simulink model "HouseExampleGood"  (R2023b)
settings: Solver=VariableStepAuto  StartTime=0.0  StopTime=3600*50  FixedStep=1  RelTol=1e-3  AbsTol=1e-3  EnableMultiTasking=on
PreLoadFcn:
  | % Walls
  | lenHouse   = 30;          % House length [m]
  | widHouse   = 10;          % House width [m]
  | htHouse     = 4;            % House height [m]
  | LWall           = 0.2;         % Wall thickness [m]
  | wallDensity = 1920;      % Density [kg/m^3]
  | c_wall          = 835;        % Specific heat [J/kg/K]
  | kWall            = 0.038;    % Thermal conductivity [W/m/K]
  | 
  | % Windows
  | n1_window       = 3;          % Number or windows in room 1
  | n2_window       = 2;          % Number or windows in room 2
  | n3_window       = 2;          % Number or windows in room 3
  | n4_window       = 2;          % Number or windows in room 4
  | htWindows       = 1;          % Height of windows [m]
  | widWindows      = 1;          % Width of windows  [m]
  | LWindow           = 0.01;     % Thickenss of windows [m]
  | windowDensity = 2700;    % Density [kg/m^3]
  | c_window          = 840;      % Specific heat [J/kg/K]
  | kWindow           = 0.78;     % Thermal conductivity [W/m/K]
  | 
  | 
  | % Roof
  | pitRoof         = 40/180/pi;   % Roof pitch (40 deg)
  | LRoof           = 0.2;             % Roof thickness [m]
  | roofDensity = 32;              % Roof density (Glass fiber) [kg/m^3]
  | c_roof          = 835;            % Specific heat [J/kg/K]
  | kRoof           = 0.038;         % Thermal conductivity [W/m/K]
  | 
  | % Radiators
  | %% Exchange area with air
  | S_radiator1 = 5;     % [m^2]
  | S_radiator2 = 5;     % [m^2]
  | S_radiator3 = 5;     % [m^2]
  | S_radiator4 = 5;     % [m^2]
  | %% Convective heat transfer coefficient radiator -> room
  | h_radiator1 = 100;  %  [W/(m^2 * K)]
  | h_radiator2 = 100;  %  [W/(m^2 * K)]
  | h_radiator3 = 100;  %  [W/(m^2 * K)]
  | h_radiator4 = 100;  %  [W/(m^2 * K)]
  | 
  | % Convective heat transfer coefficients [W/M^2/K]
  | h_air_wall         = 24;    % Indoor air->walls
  | h_wall_atm       = 34;   % Walls -> atmosphere
  | h_air_window    = 25;   % Indoor air -> windows
  | h_window_atm = 32;    % Windows -> atmosphere
  | h_air_roof         = 12;   % Indoor air -> roof
  | h_roof_atm      = 38;    % Roof -> atmosphere
  | 
  | %Air
  | c_air = 1005.4;         % cp of air at 273 K [J/(kg*K]
  | 
  | % Leakage fraction
  | leak_roof_percent = 0.1;     % Leakage through roof
  | leak_wall_percent  = 0.15;  % Leakage through walls
  | leak_win_percent  = 0.2;     % Leakage through windows
InitFcn:
  | % Roof
  | roofArea =  2* (widHouse/(2*cos(pitRoof))*lenHouse);
  | 
  | %Rooms
  | %% Room 1
  | area_window_room1 = 3 * 1 *1;
  | area_wall_room1 = (lenHouse*3/5 *htHouse+widHouse*2/3*htHouse) - area_window_room1;
  | area_roof_room1 = roofArea/4;
  | 
  | %% Room 2
  | area_window_room2 = 2 * 1 *1;
  | area_wall_room2 = (lenHouse*3/5*htHouse+widHouse/3*htHouse) - area_window_room2;
  | area_roof_room2 = roofArea/4;
  | 
  | %% Room 3
  | area_window_room3 =2* 1 *1;
  | area_wall_room3 = (lenHouse*2/5*htHouse+widHouse*2/3*htHouse) - area_window_room3;
  | area_roof_room3 = roofArea/4;
  | 
  | %% Room 4
  | area_window_room4 = 2 * 1 *1;
  | area_wall_room4 = (lenHouse*2/5*htHouse+widHouse/3*htHouse) - area_window_room4;
  | area_roof_room4 = roofArea/4;
  | 
  | % Cost estimation
  | % Assume the cost of natural gas is $8.50 per thousand cubic feet (Mcf): $8.50 per 1000 cf
  | % cost = $8.50/(1000 * 0.02831) m^3
  | cost = 8.50/(1000 * 0.02831);
  | % Natural gas density ~ 0.9 kg/m^3
  | NG_density = 0.9;
libraries: fl_lib x110, nesl_utility x11, SimscapeFluids_lib x8
(part 2 of 3)

== system HouseExampleGood/House thermal network/Radiator3 ==
  Convective Heat Transfer : fl_lib/Thermal/Thermal Elements/Convective Heat Transfer  thermal_type=foundation.enum.constant_variable.constant  area=S_radiator3 m^2  heat_tr_coeff=h_radiator3 W/(m^2 *K)  min_heat_tr_coeff=1e-3 W/(K*m^2)  T_specify=off  T_priority=None  T=0 K  T_nominal_specify=off  T_nominal_unit=K  T_nominal_value=1  Q_specify=off  Q_priority=None  Q=0 J/s  Q_nominal_specify=off  Q_nominal_unit=W  Q_nominal_value=1
  Pipe (TL) : SimscapeFluids_lib/Thermal Liquid/Pipes & Fittings/Pipe (TL)  dynamic_compressibility=1  inertia=0  num_segments=1  pipe_length=4 m  cross_section_geometry=fluids.thermal_liquid.pipes_fittings.enum.CrossSectionGeometry.Custom  pipe_diameter=0.1 m  pipe_inner_diameter=0.05 m  pipe_outer_diameter=0.1 m  pipe_width=0.1 m  pipe_height=0.1 m  pipe_major_axis=0.1 m  pipe_minor_axis=0.05 m  pipe_side=0.1 m  pipe_angle=30 deg  area=0.01 m^2  Dh=0.1128 m  elevation_spec=foundation.enum.constant_variable.constant  elevation_gain=0 m  gravity_spec=foundation.enum.constant_variable.constant  g=9.81 m/s^2  pressure_loss_spec=1  local_pressure_loss_spec=fluids.thermal_liquid.pipes_fittings.enum.LocalLossSpec.AggregateLength  length_add=1 m  loss_coefficient=0.1  roughness_spec=fluids.thermal_liquid.pipes_fittings.enum.RoughnessSpec.Custom  roughness=1.5e-5 m  Re_friction_TLU=[ 400 1000 1.5e+3 3e+3 4e+3 6e+3 1e+4 2e+4 4e+4 6e+4 1e+5 1e+8 ]  friction_factor_TLU=[ 0.264 0.112 0.07099999999999999 0.0417 0.0387 0.0268 0.025 0.0232 0.0226 0.022 0.0214 0.0214 ]  Re_lam=2e+3  Re_tur=4e+3  shape_factor=64  mdot_nominal=[ 0.1 1 ] kg/s  p_diff_nominal=[ 0.001 0.01 ] MPa  mdot_threshold=1e-6 kg/s  wall_spec=1  vol_expansion_spec=fluids.thermal_liquid.pipes_fittings.enum.VolumeExpansionSpec.Diameter  area_pressure_gain=1e-6 m^2/MPa  static_pressure_TLU=[.1, 1] MPa  area_pressure_gain_TLU=[1e-05, 1.1e-05] m^2  material_behavior_spec=fluids.thermal_liquid.pipes_fittings.enum.PipeMaterialBehavior.Linear  diameter_pressure_gain=1e-6 m/MPa  wall_thickness=0.05 m  elastic_modulus=69 GPa  stress_TLU=[276, 310] MPa  strain_TLU=[.004, .02]  stress_assert_action=simscape.enum.assert.action.none  stress_max=400 MPa  poisson_ratio=0.33  wall_time_constant=0.01 s  thermal_expansion=false  alpha_L_wall=24 um/(deltaK*m)  thermal_expansion_Tref=293.15 K  heat_transfer_spec=1  mdot_nominal_heat=[ 0.1 1 ] kg/s  T_in_nominal=[ 293.15 293.15 ] K  T_out_nominal=[ 300 300 ] K  p_in_nominal_heat=[ 0.101325 0.101325 ] MPa  T_wall_nominal=[ 303.15 303.15 ] K  a_coeff=0.023  b_Re_power=0.8  c_Pr_power=0.4  Nu_lam=3.66  Re_Colburn_TLU=[ 100 150 1000 ]  Colburn_factor_TLU=[ 0.019 0.013 0.002 ]  Re_Nu_TLU=[ 100 150 1000 ]  Pr_Nu_TLU=[ 1 10 ]  Nu_TLU=[ 3.72 4.21; 3.75 4.44; 4.21 7.15 ]  p0_vec=0.101325 MPa  T0_vec=293.15 K  mdot0=0.1 kg/s
  Radiator thermal mass : fl_lib/Thermal/Thermal Elements/Thermal Mass  mass_type=foundation.enum.constant_variable.constant  mass=46.7 kg  sp_heat=447 J/kg/K  mass_min=1e-6 kg  num_ports=foundation.enum.numPorts2.one  m_specify=off  m_priority=High  m=1 kg  m_nominal_specify=off  m_nominal_unit=kg  m_nominal_value=1  T_specify=on  T_priority=High  T=20 degC  T_nominal_specify=off  T_nominal_unit=K  T_nominal_value=1  Q_specify=off  Q_priority=High  Q=0 J/s  Q_nominal_specify=off  Q_nominal_unit=W  Q_nominal_value=1
  Inlet : PMIOPort  Side=Left
  Outlet : PMIOPort  Port=2  Side=Right
  Air : PMIOPort  Port=3  Side=Left
  connections:
  Convective Heat Transfer/RConn1 -- Air/RConn1
  Pipe (TL)/RConn1 -- Outlet/RConn1
  Pipe (TL)/LConn1 -- Inlet/RConn1
  Convective Heat Transfer/LConn1 -- Pipe (TL)/LConn2 -- Radiator thermal mass/LConn1

== system HouseExampleGood/House thermal network/Radiator4 ==
  Convective Heat Transfer : fl_lib/Thermal/Thermal Elements/Convective Heat Transfer  thermal_type=foundation.enum.constant_variable.constant  area=S_radiator4 m^2  heat_tr_coeff=h_radiator4 W/(m^2 *K)  min_heat_tr_coeff=1e-3 W/(K*m^2)  T_specify=off  T_priority=None  T=0 K  T_nominal_specify=off  T_nominal_unit=K  T_nominal_value=1  Q_specify=off  Q_priority=None  Q=0 J/s  Q_nominal_specify=off  Q_nominal_unit=W  Q_nominal_value=1
  Pipe (TL) : SimscapeFluids_lib/Thermal Liquid/Pipes & Fittings/Pipe (TL)  dynamic_compressibility=1  inertia=0  num_segments=1  pipe_length=4 m  cross_section_geometry=fluids.thermal_liquid.pipes_fittings.enum.CrossSectionGeometry.Custom  pipe_diameter=0.1 m  pipe_inner_diameter=0.05 m  pipe_outer_diameter=0.1 m  pipe_width=0.1 m  pipe_height=0.1 m  pipe_major_axis=0.1 m  pipe_minor_axis=0.05 m  pipe_side=0.1 m  pipe_angle=30 deg  area=0.01 m^2  Dh=0.1128 m  elevation_spec=foundation.enum.constant_variable.constant  elevation_gain=0 m  gravity_spec=foundation.enum.constant_variable.constant  g=9.81 m/s^2  pressure_loss_spec=1  local_pressure_loss_spec=fluids.thermal_liquid.pipes_fittings.enum.LocalLossSpec.AggregateLength  length_add=1 m  loss_coefficient=0.1  roughness_spec=fluids.thermal_liquid.pipes_fittings.enum.RoughnessSpec.Custom  roughness=1.5e-5 m  Re_friction_TLU=[ 400 1000 1.5e+3 3e+3 4e+3 6e+3 1e+4 2e+4 4e+4 6e+4 1e+5 1e+8 ]  friction_factor_TLU=[ 0.264 0.112 0.07099999999999999 0.0417 0.0387 0.0268 0.025 0.0232 0.0226 0.022 0.0214 0.0214 ]  Re_lam=2e+3  Re_tur=4e+3  shape_factor=64  mdot_nominal=[ 0.1 1 ] kg/s  p_diff_nominal=[ 0.001 0.01 ] MPa  mdot_threshold=1e-6 kg/s  wall_spec=1  vol_expansion_spec=fluids.thermal_liquid.pipes_fittings.enum.VolumeExpansionSpec.Diameter  area_pressure_gain=1e-6 m^2/MPa  static_pressure_TLU=[.1, 1] MPa  area_pressure_gain_TLU=[1e-05, 1.1e-05] m^2  material_behavior_spec=fluids.thermal_liquid.pipes_fittings.enum.PipeMaterialBehavior.Linear  diameter_pressure_gain=1e-6 m/MPa  wall_thickness=0.05 m  elastic_modulus=69 GPa  stress_TLU=[276, 310] MPa  strain_TLU=[.004, .02]  stress_assert_action=simscape.enum.assert.action.none  stress_max=400 MPa  poisson_ratio=0.33  wall_time_constant=0.01 s  thermal_expansion=false  alpha_L_wall=24 um/(deltaK*m)  thermal_expansion_Tref=293.15 K  heat_transfer_spec=1  mdot_nominal_heat=[ 0.1 1 ] kg/s  T_in_nominal=[ 293.15 293.15 ] K  T_out_nominal=[ 300 300 ] K  p_in_nominal_heat=[ 0.101325 0.101325 ] MPa  T_wall_nominal=[ 303.15 303.15 ] K  a_coeff=0.023  b_Re_power=0.8  c_Pr_power=0.4  Nu_lam=3.66  Re_Colburn_TLU=[ 100 150 1000 ]  Colburn_factor_TLU=[ 0.019 0.013 0.002 ]  Re_Nu_TLU=[ 100 150 1000 ]  Pr_Nu_TLU=[ 1 10 ]  Nu_TLU=[ 3.72 4.21; 3.75 4.44; 4.21 7.15 ]  p0_vec=0.101325 MPa  T0_vec=293.15 K  mdot0=0.1 kg/s
  Radiator thermal mass : fl_lib/Thermal/Thermal Elements/Thermal Mass  mass_type=foundation.enum.constant_variable.constant  mass=46.7 kg  sp_heat=447 J/kg/K  mass_min=1e-6 kg  num_ports=foundation.enum.numPorts2.one  m_specify=off  m_priority=High  m=1 kg  m_nominal_specify=off  m_nominal_unit=kg  m_nominal_value=1  T_specify=on  T_priority=High  T=20 degC  T_nominal_specify=off  T_nominal_unit=K  T_nominal_value=1  Q_specify=off  Q_priority=High  Q=0 J/s  Q_nominal_specify=off  Q_nominal_unit=W  Q_nominal_value=1
  Inlet : PMIOPort  Side=Left
  Outlet : PMIOPort  Port=2  Side=Right
  Air : PMIOPort  Port=3  Side=Left
  connections:
  Radiator thermal mass/LConn1 -- Pipe (TL)/LConn2 -- Convective Heat Transfer/LConn1
  Pipe (TL)/LConn1 -- Inlet/RConn1
  Pipe (TL)/RConn1 -- Outlet/RConn1
  Convective Heat Transfer/RConn1 -- Air/RConn1

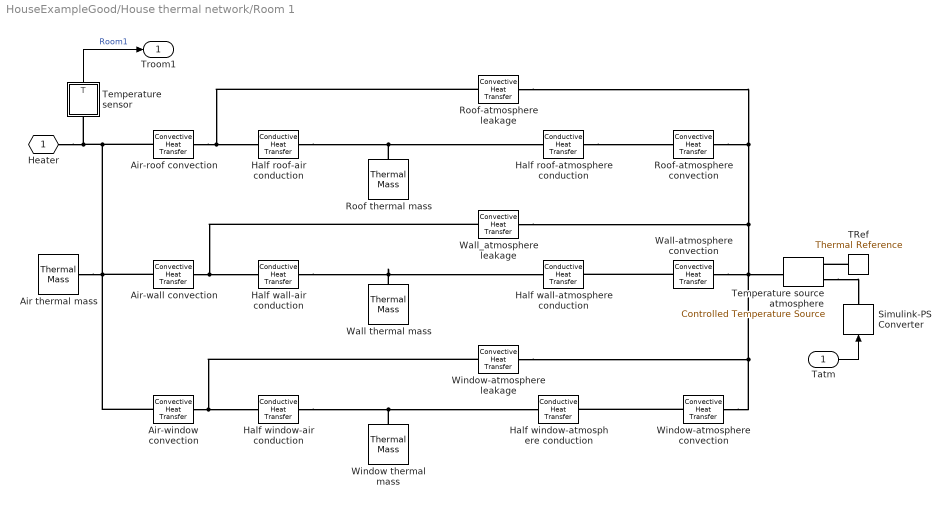
== system HouseExampleGood/House thermal network/Room 1 ==
  Tatm : Inport
  Air thermal mass : fl_lib/Thermal/Thermal Elements/Thermal Mass  mass_type=foundation.enum.constant_variable.constant  mass=50 kg  sp_heat=c_air J/kg/K  mass_min=1e-6 kg  num_ports=foundation.enum.numPorts2.one  m_specify=off  m_priority=High  m=1 kg  m_nominal_specify=off  m_nominal_unit=kg  m_nominal_value=1  T_specify=on  T_priority=High  T=20 degC  T_nominal_specify=off  T_nominal_unit=K  T_nominal_value=1  Q_specify=off  Q_priority=High  Q=0 J/s  Q_nominal_specify=off  Q_nominal_unit=W  Q_nominal_value=1
  Air-roof convection : fl_lib/Thermal/Thermal Elements/Convective Heat Transfer  thermal_type=foundation.enum.constant_variable.constant  area=area_roof_room1 m^2  heat_tr_coeff=h_air_roof W/(m^2 * K)  min_heat_tr_coeff=1e-3 W/(K*m^2)  T_specify=off  T_priority=None  T=0 K  T_nominal_specify=off  T_nominal_unit=K  T_nominal_value=1  Q_specify=off  Q_priority=None  Q=0 J/s  Q_nominal_specify=off  Q_nominal_unit=W  Q_nominal_value=1
  Air-wall convection : fl_lib/Thermal/Thermal Elements/Convective Heat Transfer  thermal_type=foundation.enum.constant_variable.constant  area=area_wall_room1 m^2  heat_tr_coeff=h_air_wall W/(m^2 * K)  min_heat_tr_coeff=1e-3 W/(K*m^2)  T_specify=off  T_priority=None  T=0 K  T_nominal_specify=off  T_nominal_unit=K  T_nominal_value=1  Q_specify=off  Q_priority=None  Q=0 J/s  Q_nominal_specify=off  Q_nominal_unit=W  Q_nominal_value=1
  Air-window convection : fl_lib/Thermal/Thermal Elements/Convective Heat Transfer  thermal_type=foundation.enum.constant_variable.constant  area=area_window_room1 m^2  heat_tr_coeff=h_air_window W/(m^2 * K)  min_heat_tr_coeff=1e-3 W/(K*m^2)  T_specify=off  T_priority=None  T=0 K  T_nominal_specify=off  T_nominal_unit=K  T_nominal_value=1  Q_specify=off  Q_priority=None  Q=0 J/s  Q_nominal_specify=off  Q_nominal_unit=W  Q_nominal_value=1
  Half roof-air conduction : fl_lib/Thermal/Thermal Elements/Conductive Heat Transfer  thermal_type=foundation.enum.ConstantVariableTabulated.Constant  wall_geometry=foundation.enum.ConductionWallGeometry.Planar  area=area_roof_room1 m^2  thickness=LRoof/2 m  d_in=0.05 m  d_out=0.1 m  L=1 m  th_cond_min=10 W/(K*m)  th_cond=kRoof W/(m*K)  th_cond_TLU=[413, 401, 392, 383, 371, 357, 342] W/(K*m)  temp_TLU=[200, 273, 400, 600, 800, 1000, 1200] K  T_specify=off  T_priority=None  T=0 K  T_nominal_specify=off  T_nominal_unit=K  T_nominal_value=1  Q_specify=off  Q_priority=None  Q=0 J/s  Q_nominal_specify=off  Q_nominal_unit=W  Q_nominal_value=1
  Half roof-atmosphere conduction : fl_lib/Thermal/Thermal Elements/Conductive Heat Transfer  thermal_type=foundation.enum.ConstantVariableTabulated.Constant  wall_geometry=foundation.enum.ConductionWallGeometry.Planar  area=area_roof_room1 m^2  thickness=LRoof/2 m  d_in=0.05 m  d_out=0.1 m  L=1 m  th_cond_min=10 W/(K*m)  th_cond=kRoof W/(m*K)  th_cond_TLU=[413, 401, 392, 383, 371, 357, 342] W/(K*m)  temp_TLU=[200, 273, 400, 600, 800, 1000, 1200] K  T_specify=off  T_priority=None  T=0 K  T_nominal_specify=off  T_nominal_unit=K  T_nominal_value=1  Q_specify=off  Q_priority=None  Q=0 J/s  Q_nominal_specify=off  Q_nominal_unit=W  Q_nominal_value=1
  Half wall-air conduction : fl_lib/Thermal/Thermal Elements/Conductive Heat Transfer  thermal_type=foundation.enum.ConstantVariableTabulated.Constant  wall_geometry=foundation.enum.ConductionWallGeometry.Planar  area=area_wall_room1 m^2  thickness=LWall/2 m  d_in=0.05 m  d_out=0.1 m  L=1 m  th_cond_min=10 W/(K*m)  th_cond=kWall W/(m*K)  th_cond_TLU=[413, 401, 392, 383, 371, 357, 342] W/(K*m)  temp_TLU=[200, 273, 400, 600, 800, 1000, 1200] K  T_specify=off  T_priority=None  T=0 K  T_nominal_specify=off  T_nominal_unit=K  T_nominal_value=1  Q_specify=off  Q_priority=None  Q=0 J/s  Q_nominal_specify=off  Q_nominal_unit=W  Q_nominal_value=1
  Half wall-atmosphere conduction : fl_lib/Thermal/Thermal Elements/Conductive Heat Transfer  thermal_type=foundation.enum.ConstantVariableTabulated.Constant  wall_geometry=foundation.enum.ConductionWallGeometry.Planar  area=area_wall_room1 m^2  thickness=LWall/2 m  d_in=0.05 m  d_out=0.1 m  L=1 m  th_cond_min=10 W/(K*m)  th_cond=kWall W/(m*K)  th_cond_TLU=[413, 401, 392, 383, 371, 357, 342] W/(K*m)  temp_TLU=[200, 273, 400, 600, 800, 1000, 1200] K  T_specify=off  T_priority=None  T=0 K  T_nominal_specify=off  T_nominal_unit=K  T_nominal_value=1  Q_specify=off  Q_priority=None  Q=0 J/s  Q_nominal_specify=off  Q_nominal_unit=W  Q_nominal_value=1
  Half window-air conduction : fl_lib/Thermal/Thermal Elements/Conductive Heat Transfer  thermal_type=foundation.enum.ConstantVariableTabulated.Constant  wall_geometry=foundation.enum.ConductionWallGeometry.Planar  area=area_window_room1 m^2  thickness=LWindow/2 m  d_in=0.05 m  d_out=0.1 m  L=1 m  th_cond_min=10 W/(K*m)  th_cond=kWindow W/(m*K)  th_cond_TLU=[413, 401, 392, 383, 371, 357, 342] W/(K*m)  temp_TLU=[200, 273, 400, 600, 800, 1000, 1200] K  T_specify=off  T_priority=None  T=0 K  T_nominal_specify=off  T_nominal_unit=K  T_nominal_value=1  Q_specify=off  Q_priority=None  Q=0 J/s  Q_nominal_specify=off  Q_nominal_unit=W  Q_nominal_value=1
  Half window-atmosphere conduction : fl_lib/Thermal/Thermal Elements/Conductive Heat Transfer  thermal_type=foundation.enum.ConstantVariableTabulated.Constant  wall_geometry=foundation.enum.ConductionWallGeometry.Planar  area=area_window_room1 m^2  thickness=LWindow/2 m  d_in=0.05 m  d_out=0.1 m  L=1 m  th_cond_min=10 W/(K*m)  th_cond=kWindow W/(m*K)  th_cond_TLU=[413, 401, 392, 383, 371, 357, 342] W/(K*m)  temp_TLU=[200, 273, 400, 600, 800, 1000, 1200] K  T_specify=off  T_priority=None  T=0 K  T_nominal_specify=off  T_nominal_unit=K  T_nominal_value=1  Q_specify=off  Q_priority=None  Q=0 J/s  Q_nominal_specify=off  Q_nominal_unit=W  Q_nominal_value=1
  Roof thermal mass : fl_lib/Thermal/Thermal Elements/Thermal Mass  mass_type=foundation.enum.constant_variable.constant  mass=area_roof_room1*LRoof*roofDensity kg  sp_heat=c_roof J/kg/K  mass_min=1e-6 kg  num_ports=foundation.enum.numPorts2.one  m_specify=off  m_priority=High  m=1 kg  m_nominal_specify=off  m_nominal_unit=kg  m_nominal_value=1  T_specify=on  T_priority=High  T=20 degC  T_nominal_specify=off  T_nominal_unit=K  T_nominal_value=1  Q_specify=off  Q_priority=None  Q=0 J/s  Q_nominal_specify=off  Q_nominal_unit=W  Q_nominal_value=1
  Roof-atmosphere convection : fl_lib/Thermal/Thermal Elements/Convective Heat Transfer  thermal_type=foundation.enum.constant_variable.constant  area=area_roof_room1 m^2  heat_tr_coeff=h_roof_atm W/(m^2 * K)  min_heat_tr_coeff=1e-3 W/(K*m^2)  T_specify=off  T_priority=None  T=0 K  T_nominal_specify=off  T_nominal_unit=K  T_nominal_value=1  Q_specify=off  Q_priority=None  Q=0 J/s  Q_nominal_specify=off  Q_nominal_unit=W  Q_nominal_value=1
  Roof-atmosphere leakage : fl_lib/Thermal/Thermal Elements/Convective Heat Transfer  thermal_type=foundation.enum.constant_variable.constant  area=area_roof_room1*leak_roof_percent m^2  heat_tr_coeff=h_roof_atm W/(m^2 * K)  min_heat_tr_coeff=1e-3 W/(K*m^2)  T_specify=off  T_priority=None  T=0 K  T_nominal_specify=off  T_nominal_unit=K  T_nominal_value=1  Q_specify=off  Q_priority=None  Q=0 J/s  Q_nominal_specify=off  Q_nominal_unit=W  Q_nominal_value=1
  Simulink-PS Converter : nesl_utility/Simulink-PS Converter  PhysicalDomain=network_engine_domain  SubClassName=ps_input  LeftPortType=input  RightPortType=output  PseudoPeriodic=off  Frequencies=[]  NoiseDistribution=none  NoiseParameters=[]  Unit=degC  AffineConversion=on  FilteringAndDerivatives=zero  SimscapeFilterOrder=1  InputFilterTimeConstant=.001  UdotUserProvided=1
  TRef : fl_lib/Thermal/Thermal Elements/Thermal Reference
  Temperature source atmosphere : fl_lib/Thermal/Thermal Sources/Controlled Temperature Source
  Temperature sensor : Subsystem
  Wall thermal mass : fl_lib/Thermal/Thermal Elements/Thermal Mass  mass_type=foundation.enum.constant_variable.constant  mass=area_wall_room1 * LWall * wallDensity kg  sp_heat=c_wall J/kg/K  mass_min=1e-6 kg  num_ports=foundation.enum.numPorts2.one  m_specify=off  m_priority=High  m=1 kg  m_nominal_specify=off  m_nominal_unit=kg  m_nominal_value=1  T_specify=on  T_priority=High  T=20 degC  T_nominal_specify=off  T_nominal_unit=K  T_nominal_value=1  Q_specify=off  Q_priority=None  Q=0 J/s  Q_nominal_specify=off  Q_nominal_unit=W  Q_nominal_value=1
  Wall-atmosphere convection : fl_lib/Thermal/Thermal Elements/Convective Heat Transfer  thermal_type=foundation.enum.constant_variable.constant  area=area_wall_room1 m^2  heat_tr_coeff=h_wall_atm W/(m^2 * K)  min_heat_tr_coeff=1e-3 W/(K*m^2)  T_specify=off  T_priority=None  T=0 K  T_nominal_specify=off  T_nominal_unit=K  T_nominal_value=1  Q_specify=off  Q_priority=None  Q=0 J/s  Q_nominal_specify=off  Q_nominal_unit=W  Q_nominal_value=1
  Wall_atmosphere leakage : fl_lib/Thermal/Thermal Elements/Convective Heat Transfer  thermal_type=foundation.enum.constant_variable.constant  area=area_wall_room1*leak_wall_percent m^2  heat_tr_coeff=h_wall_atm W/(m^2 * K)  min_heat_tr_coeff=1e-3 W/(K*m^2)  T_specify=off  T_priority=None  T=0 K  T_nominal_specify=off  T_nominal_unit=K  T_nominal_value=1  Q_specify=off  Q_priority=None  Q=0 J/s  Q_nominal_specify=off  Q_nominal_unit=W  Q_nominal_value=1
  Window thermal mass : fl_lib/Thermal/Thermal Elements/Thermal Mass  mass_type=foundation.enum.constant_variable.constant  mass=area_window_room1 * LWindow * windowDensity kg  sp_heat=c_window J/kg/K  mass_min=1e-6 kg  num_ports=foundation.enum.numPorts2.one  m_specify=off  m_priority=High  m=1 kg  m_nominal_specify=off  m_nominal_unit=kg  m_nominal_value=1  T_specify=on  T_priority=High  T=20 degC  T_nominal_specify=off  T_nominal_unit=K  T_nominal_value=1  Q_specify=off  Q_priority=None  Q=0 J/s  Q_nominal_specify=off  Q_nominal_unit=W  Q_nominal_value=1
  Window-atmosphere convection : fl_lib/Thermal/Thermal Elements/Convective Heat Transfer  thermal_type=foundation.enum.constant_variable.constant  area=area_window_room1 m^2  heat_tr_coeff=h_window_atm W/(m^2 * K)  min_heat_tr_coeff=1e-3 W/(K*m^2)  T_specify=off  T_priority=None  T=0 K  T_nominal_specify=off  T_nominal_unit=K  T_nominal_value=1  Q_specify=off  Q_priority=None  Q=0 J/s  Q_nominal_specify=off  Q_nominal_unit=W  Q_nominal_value=1
  Window-atmosphere leakage : fl_lib/Thermal/Thermal Elements/Convective Heat Transfer  thermal_type=foundation.enum.constant_variable.constant  area=area_window_room1*leak_win_percent m^2  heat_tr_coeff=h_window_atm W/(m^2 * K)  min_heat_tr_coeff=1e-3 W/(K*m^2)  T_specify=off  T_priority=None  T=0 K  T_nominal_specify=off  T_nominal_unit=K  T_nominal_value=1  Q_specify=off  Q_priority=None  Q=0 J/s  Q_nominal_specify=off  Q_nominal_unit=W  Q_nominal_value=1
  Heater : PMIOPort  Tag=PMCPort  Side=Left
  Troom1 : Outport  VectorParamsAs1DForOutWhenUnconnected=off
  wires:
  Temperature sensor/1(T) -> Troom1/1  "Room1"
  Tatm/1 -> Simulink-PS Converter/1
  connections:
  Temperature sensor/LConn1 -- Air-window convection/LConn1 -- Air thermal mass/LConn1 -- Air-wall convection/LConn1 -- Air-roof convection/LConn1 -- Heater/RConn1
  TRef/LConn1 -- Temperature source atmosphere/RConn2
  Half wall-air conduction/RConn1 -- Half wall-atmosphere conduction/LConn1 -- Wall thermal mass/LConn1
  Half window-air conduction/RConn1 -- Window thermal mass/LConn1 -- Half window-atmosphere conduction/LConn1
  Half roof-air conduction/RConn1 -- Half roof-atmosphere conduction/LConn1 -- Roof thermal mass/LConn1
  Air-wall convection/RConn1 -- Wall_atmosphere leakage/LConn1 -- Half wall-air conduction/LConn1
  Air-window convection/RConn1 -- Window-atmosphere leakage/LConn1 -- Half window-air conduction/LConn1
  Wall-atmosphere convection/LConn1 -- Half wall-atmosphere conduction/RConn1
  Window-atmosphere convection/LConn1 -- Half window-atmosphere conduction/RConn1
  Air-roof convection/RConn1 -- Roof-atmosphere leakage/LConn1 -- Half roof-air conduction/LConn1
  Temperature source atmosphere/RConn1 -- Simulink-PS Converter/RConn1
  Half roof-atmosphere conduction/RConn1 -- Roof-atmosphere convection/LConn1
  Wall-atmosphere convection/RConn1 -- Window-atmosphere leakage/RConn1 -- Window-atmosphere convection/RConn1 -- Wall_atmosphere leakage/RConn1 -- Roof-atmosphere convection/RConn1 -- Roof-atmosphere leakage/RConn1 -- Temperature source atmosphere/LConn1

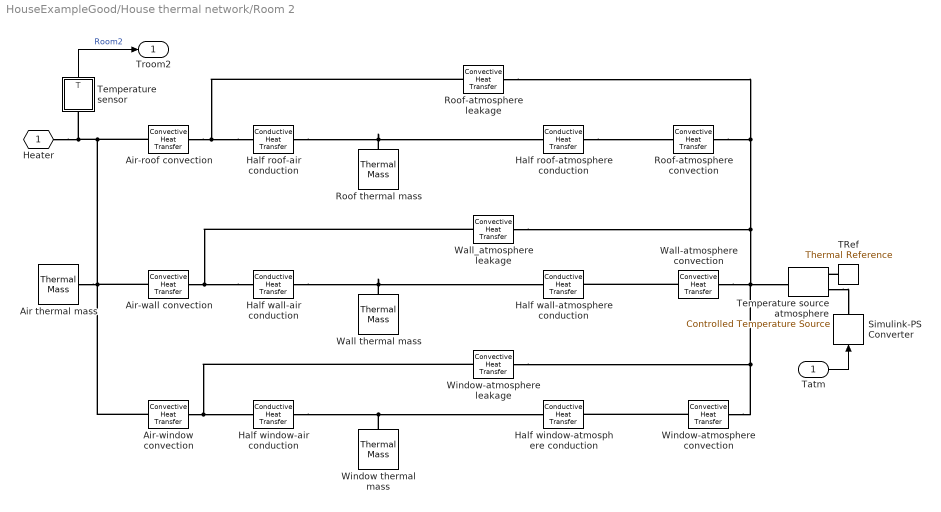
== system HouseExampleGood/House thermal network/Room 2 ==
  Tatm : Inport
  Air thermal mass : fl_lib/Thermal/Thermal Elements/Thermal Mass  mass_type=foundation.enum.constant_variable.constant  mass=50 kg  sp_heat=c_air J/kg/K  mass_min=1e-6 kg  num_ports=foundation.enum.numPorts2.one  m_specify=off  m_priority=High  m=1 kg  m_nominal_specify=off  m_nominal_unit=kg  m_nominal_value=1  T_specify=on  T_priority=High  T=20 degC  T_nominal_specify=off  T_nominal_unit=K  T_nominal_value=1  Q_specify=off  Q_priority=High  Q=0 J/s  Q_nominal_specify=off  Q_nominal_unit=W  Q_nominal_value=1
  Air-roof convection : fl_lib/Thermal/Thermal Elements/Convective Heat Transfer  thermal_type=foundation.enum.constant_variable.constant  area=area_roof_room2 m^2  heat_tr_coeff=h_air_roof W/(m^2 * K)  min_heat_tr_coeff=1e-3 W/(K*m^2)  T_specify=off  T_priority=None  T=0 K  T_nominal_specify=off  T_nominal_unit=K  T_nominal_value=1  Q_specify=off  Q_priority=None  Q=0 J/s  Q_nominal_specify=off  Q_nominal_unit=W  Q_nominal_value=1
  Air-wall convection : fl_lib/Thermal/Thermal Elements/Convective Heat Transfer  thermal_type=foundation.enum.constant_variable.constant  area=area_wall_room2 m^2  heat_tr_coeff=h_air_wall W/(m^2 * K)  min_heat_tr_coeff=1e-3 W/(K*m^2)  T_specify=off  T_priority=None  T=0 K  T_nominal_specify=off  T_nominal_unit=K  T_nominal_value=1  Q_specify=off  Q_priority=None  Q=0 J/s  Q_nominal_specify=off  Q_nominal_unit=W  Q_nominal_value=1
  Air-window convection : fl_lib/Thermal/Thermal Elements/Convective Heat Transfer  thermal_type=foundation.enum.constant_variable.constant  area=area_window_room2 m^2  heat_tr_coeff=h_air_window W/(m^2 * K)  min_heat_tr_coeff=1e-3 W/(K*m^2)  T_specify=off  T_priority=None  T=0 K  T_nominal_specify=off  T_nominal_unit=K  T_nominal_value=1  Q_specify=off  Q_priority=None  Q=0 J/s  Q_nominal_specify=off  Q_nominal_unit=W  Q_nominal_value=1
  Half roof-air conduction : fl_lib/Thermal/Thermal Elements/Conductive Heat Transfer  thermal_type=foundation.enum.ConstantVariableTabulated.Constant  wall_geometry=foundation.enum.ConductionWallGeometry.Planar  area=area_roof_room2 m^2  thickness=LRoof/2 m  d_in=0.05 m  d_out=0.1 m  L=1 m  th_cond_min=10 W/(K*m)  th_cond=kRoof W/(m*K)  th_cond_TLU=[413, 401, 392, 383, 371, 357, 342] W/(K*m)  temp_TLU=[200, 273, 400, 600, 800, 1000, 1200] K  T_specify=off  T_priority=None  T=0 K  T_nominal_specify=off  T_nominal_unit=K  T_nominal_value=1  Q_specify=off  Q_priority=None  Q=0 J/s  Q_nominal_specify=off  Q_nominal_unit=W  Q_nominal_value=1
  Half roof-atmosphere conduction : fl_lib/Thermal/Thermal Elements/Conductive Heat Transfer  thermal_type=foundation.enum.ConstantVariableTabulated.Constant  wall_geometry=foundation.enum.ConductionWallGeometry.Planar  area=area_roof_room2 m^2  thickness=LRoof/2 m  d_in=0.05 m  d_out=0.1 m  L=1 m  th_cond_min=10 W/(K*m)  th_cond=kRoof W/(m*K)  th_cond_TLU=[413, 401, 392, 383, 371, 357, 342] W/(K*m)  temp_TLU=[200, 273, 400, 600, 800, 1000, 1200] K  T_specify=off  T_priority=None  T=0 K  T_nominal_specify=off  T_nominal_unit=K  T_nominal_value=1  Q_specify=off  Q_priority=None  Q=0 J/s  Q_nominal_specify=off  Q_nominal_unit=W  Q_nominal_value=1
  Half wall-air conduction : fl_lib/Thermal/Thermal Elements/Conductive Heat Transfer  thermal_type=foundation.enum.ConstantVariableTabulated.Constant  wall_geometry=foundation.enum.ConductionWallGeometry.Planar  area=area_wall_room2 m^2  thickness=LWall/2 m  d_in=0.05 m  d_out=0.1 m  L=1 m  th_cond_min=10 W/(K*m)  th_cond=kWall W/(m*K)  th_cond_TLU=[413, 401, 392, 383, 371, 357, 342] W/(K*m)  temp_TLU=[200, 273, 400, 600, 800, 1000, 1200] K  T_specify=off  T_priority=None  T=0 K  T_nominal_specify=off  T_nominal_unit=K  T_nominal_value=1  Q_specify=off  Q_priority=None  Q=0 J/s  Q_nominal_specify=off  Q_nominal_unit=W  Q_nominal_value=1
  Half wall-atmosphere conduction : fl_lib/Thermal/Thermal Elements/Conductive Heat Transfer  thermal_type=foundation.enum.ConstantVariableTabulated.Constant  wall_geometry=foundation.enum.ConductionWallGeometry.Planar  area=area_wall_room2 m^2  thickness=LWall/2 m  d_in=0.05 m  d_out=0.1 m  L=1 m  th_cond_min=10 W/(K*m)  th_cond=kWall W/(m*K)  th_cond_TLU=[413, 401, 392, 383, 371, 357, 342] W/(K*m)  temp_TLU=[200, 273, 400, 600, 800, 1000, 1200] K  T_specify=off  T_priority=None  T=0 K  T_nominal_specify=off  T_nominal_unit=K  T_nominal_value=1  Q_specify=off  Q_priority=None  Q=0 J/s  Q_nominal_specify=off  Q_nominal_unit=W  Q_nominal_value=1
  Half window-air conduction : fl_lib/Thermal/Thermal Elements/Conductive Heat Transfer  thermal_type=foundation.enum.ConstantVariableTabulated.Constant  wall_geometry=foundation.enum.ConductionWallGeometry.Planar  area=area_window_room2 m^2  thickness=LWindow/2 m  d_in=0.05 m  d_out=0.1 m  L=1 m  th_cond_min=10 W/(K*m)  th_cond=kWindow W/(m*K)  th_cond_TLU=[413, 401, 392, 383, 371, 357, 342] W/(K*m)  temp_TLU=[200, 273, 400, 600, 800, 1000, 1200] K  T_specify=off  T_priority=None  T=0 K  T_nominal_specify=off  T_nominal_unit=K  T_nominal_value=1  Q_specify=off  Q_priority=None  Q=0 J/s  Q_nominal_specify=off  Q_nominal_unit=W  Q_nominal_value=1
  Half window-atmosphere conduction : fl_lib/Thermal/Thermal Elements/Conductive Heat Transfer  thermal_type=foundation.enum.ConstantVariableTabulated.Constant  wall_geometry=foundation.enum.ConductionWallGeometry.Planar  area=area_window_room2 m^2  thickness=LWindow/2 m  d_in=0.05 m  d_out=0.1 m  L=1 m  th_cond_min=10 W/(K*m)  th_cond=kWindow W/(m*K)  th_cond_TLU=[413, 401, 392, 383, 371, 357, 342] W/(K*m)  temp_TLU=[200, 273, 400, 600, 800, 1000, 1200] K  T_specify=off  T_priority=None  T=0 K  T_nominal_specify=off  T_nominal_unit=K  T_nominal_value=1  Q_specify=off  Q_priority=None  Q=0 J/s  Q_nominal_specify=off  Q_nominal_unit=W  Q_nominal_value=1
  Roof thermal mass : fl_lib/Thermal/Thermal Elements/Thermal Mass  mass_type=foundation.enum.constant_variable.constant  mass=area_roof_room2*LRoof*roofDensity kg  sp_heat=c_roof J/kg/K  mass_min=1e-6 kg  num_ports=foundation.enum.numPorts2.one  m_specify=off  m_priority=High  m=1 kg  m_nominal_specify=off  m_nominal_unit=kg  m_nominal_value=1  T_specify=on  T_priority=High  T=20 degC  T_nominal_specify=off  T_nominal_unit=K  T_nominal_value=1  Q_specify=off  Q_priority=None  Q=0 J/s  Q_nominal_specify=off  Q_nominal_unit=W  Q_nominal_value=1
  Roof-atmosphere convection : fl_lib/Thermal/Thermal Elements/Convective Heat Transfer  thermal_type=foundation.enum.constant_variable.constant  area=area_roof_room2 m^2  heat_tr_coeff=h_roof_atm W/(m^2 * K)  min_heat_tr_coeff=1e-3 W/(K*m^2)  T_specify=off  T_priority=None  T=0 K  T_nominal_specify=off  T_nominal_unit=K  T_nominal_value=1  Q_specify=off  Q_priority=None  Q=0 J/s  Q_nominal_specify=off  Q_nominal_unit=W  Q_nominal_value=1
  Roof-atmosphere leakage : fl_lib/Thermal/Thermal Elements/Convective Heat Transfer  thermal_type=foundation.enum.constant_variable.constant  area=area_roof_room2*leak_roof_percent m^2  heat_tr_coeff=h_roof_atm W/(m^2 * K)  min_heat_tr_coeff=1e-3 W/(K*m^2)  T_specify=off  T_priority=None  T=0 K  T_nominal_specify=off  T_nominal_unit=K  T_nominal_value=1  Q_specify=off  Q_priority=None  Q=0 J/s  Q_nominal_specify=off  Q_nominal_unit=W  Q_nominal_value=1
  Simulink-PS Converter : nesl_utility/Simulink-PS Converter  PhysicalDomain=network_engine_domain  SubClassName=ps_input  LeftPortType=input  RightPortType=output  PseudoPeriodic=off  Frequencies=[]  NoiseDistribution=none  NoiseParameters=[]  Unit=degC  AffineConversion=on  FilteringAndDerivatives=zero  SimscapeFilterOrder=1  InputFilterTimeConstant=.001  UdotUserProvided=1
  TRef : fl_lib/Thermal/Thermal Elements/Thermal Reference
  Temperature source atmosphere : fl_lib/Thermal/Thermal Sources/Controlled Temperature Source
  Temperature sensor : Subsystem
  Wall thermal mass : fl_lib/Thermal/Thermal Elements/Thermal Mass  mass_type=foundation.enum.constant_variable.constant  mass=area_wall_room2 * LWall * wallDensity kg  sp_heat=c_wall J/kg/K  mass_min=1e-6 kg  num_ports=foundation.enum.numPorts2.one  m_specify=off  m_priority=High  m=1 kg  m_nominal_specify=off  m_nominal_unit=kg  m_nominal_value=1  T_specify=on  T_priority=High  T=20 degC  T_nominal_specify=off  T_nominal_unit=K  T_nominal_value=1  Q_specify=off  Q_priority=None  Q=0 J/s  Q_nominal_specify=off  Q_nominal_unit=W  Q_nominal_value=1
  Wall-atmosphere convection : fl_lib/Thermal/Thermal Elements/Convective Heat Transfer  thermal_type=foundation.enum.constant_variable.constant  area=area_wall_room2 m^2  heat_tr_coeff=h_wall_atm W/(m^2 * K)  min_heat_tr_coeff=1e-3 W/(K*m^2)  T_specify=off  T_priority=None  T=0 K  T_nominal_specify=off  T_nominal_unit=K  T_nominal_value=1  Q_specify=off  Q_priority=None  Q=0 J/s  Q_nominal_specify=off  Q_nominal_unit=W  Q_nominal_value=1
  Wall_atmosphere leakage : fl_lib/Thermal/Thermal Elements/Convective Heat Transfer  thermal_type=foundation.enum.constant_variable.constant  area=area_wall_room2*leak_wall_percent m^2  heat_tr_coeff=h_wall_atm W/(m^2 * K)  min_heat_tr_coeff=1e-3 W/(K*m^2)  T_specify=off  T_priority=None  T=0 K  T_nominal_specify=off  T_nominal_unit=K  T_nominal_value=1  Q_specify=off  Q_priority=None  Q=0 J/s  Q_nominal_specify=off  Q_nominal_unit=W  Q_nominal_value=1
  Window thermal mass : fl_lib/Thermal/Thermal Elements/Thermal Mass  mass_type=foundation.enum.constant_variable.constant  mass=area_window_room2 * LWindow * windowDensity kg  sp_heat=c_window J/kg/K  mass_min=1e-6 kg  num_ports=foundation.enum.numPorts2.one  m_specify=off  m_priority=High  m=1 kg  m_nominal_specify=off  m_nominal_unit=kg  m_nominal_value=1  T_specify=on  T_priority=High  T=20 degC  T_nominal_specify=off  T_nominal_unit=K  T_nominal_value=1  Q_specify=off  Q_priority=None  Q=0 J/s  Q_nominal_specify=off  Q_nominal_unit=W  Q_nominal_value=1
  Window-atmosphere convection : fl_lib/Thermal/Thermal Elements/Convective Heat Transfer  thermal_type=foundation.enum.constant_variable.constant  area=area_window_room2 m^2  heat_tr_coeff=h_window_atm W/(m^2 * K)  min_heat_tr_coeff=1e-3 W/(K*m^2)  T_specify=off  T_priority=None  T=0 K  T_nominal_specify=off  T_nominal_unit=K  T_nominal_value=1  Q_specify=off  Q_priority=None  Q=0 J/s  Q_nominal_specify=off  Q_nominal_unit=W  Q_nominal_value=1
  Window-atmosphere leakage : fl_lib/Thermal/Thermal Elements/Convective Heat Transfer  thermal_type=foundation.enum.constant_variable.constant  area=area_window_room2*leak_win_percent m^2  heat_tr_coeff=h_window_atm W/(m^2 * K)  min_heat_tr_coeff=1e-3 W/(K*m^2)  T_specify=off  T_priority=None  T=0 K  T_nominal_specify=off  T_nominal_unit=K  T_nominal_value=1  Q_specify=off  Q_priority=None  Q=0 J/s  Q_nominal_specify=off  Q_nominal_unit=W  Q_nominal_value=1
  Heater : PMIOPort  Tag=PMCPort  Side=Left
  Troom2 : Outport  VectorParamsAs1DForOutWhenUnconnected=off
  wires:
  Temperature sensor/1(T) -> Troom2/1  "Room2"
  Tatm/1 -> Simulink-PS Converter/1
  connections:
  Air-roof convection/LConn1 -- Air thermal mass/LConn1 -- Air-wall convection/LConn1 -- Air-window convection/LConn1 -- Heater/RConn1 -- Temperature sensor/LConn1
  Wall thermal mass/LConn1 -- Half wall-atmosphere conduction/LConn1 -- Half wall-air conduction/RConn1
  Window thermal mass/LConn1 -- Half window-atmosphere conduction/LConn1 -- Half window-air conduction/RConn1
  Roof thermal mass/LConn1 -- Half roof-atmosphere conduction/LConn1 -- Half roof-air conduction/RConn1
  Wall-atmosphere convection/RConn1 -- Window-atmosphere leakage/RConn1 -- Window-atmosphere convection/RConn1 -- Roof-atmosphere leakage/RConn1 -- Roof-atmosphere convection/RConn1 -- Wall_atmosphere leakage/RConn1 -- Temperature source atmosphere/LConn1
  Half wall-air conduction/LConn1 -- Air-wall convection/RConn1 -- Wall_atmosphere leakage/LConn1
  Air-window convection/RConn1 -- Window-atmosphere leakage/LConn1 -- Half window-air conduction/LConn1
  Half roof-air conduction/LConn1 -- Air-roof convection/RConn1 -- Roof-atmosphere leakage/LConn1
  Wall-atmosphere convection/LConn1 -- Half wall-atmosphere conduction/RConn1
  Window-atmosphere convection/LConn1 -- Half window-atmosphere conduction/RConn1
  Half roof-atmosphere conduction/RConn1 -- Roof-atmosphere convection/LConn1
  TRef/LConn1 -- Temperature source atmosphere/RConn2
  Temperature source atmosphere/RConn1 -- Simulink-PS Converter/RConn1

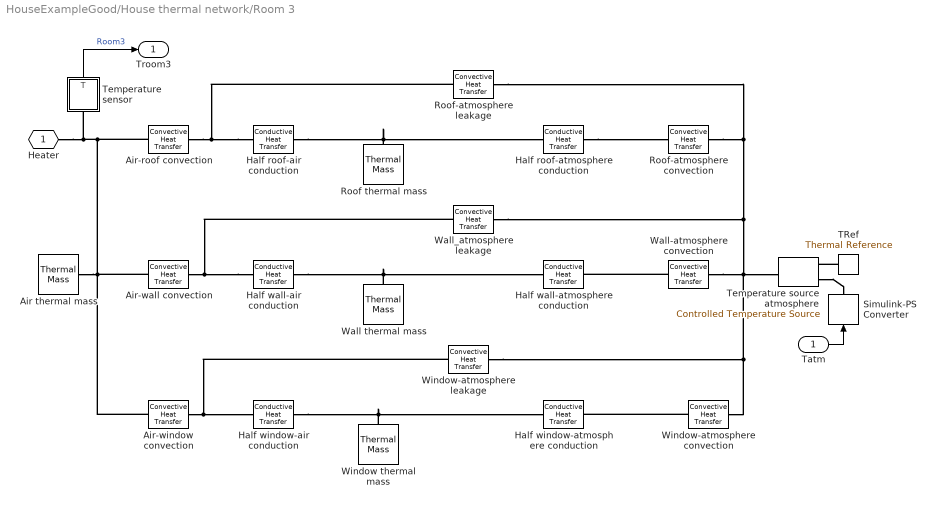
== system HouseExampleGood/House thermal network/Room 3 ==
  Tatm : Inport
  Air thermal mass : fl_lib/Thermal/Thermal Elements/Thermal Mass  mass_type=foundation.enum.constant_variable.constant  mass=50 kg  sp_heat=c_air J/kg/K  mass_min=1e-6 kg  num_ports=foundation.enum.numPorts2.one  m_specify=off  m_priority=High  m=1 kg  m_nominal_specify=off  m_nominal_unit=kg  m_nominal_value=1  T_specify=on  T_priority=High  T=20 degC  T_nominal_specify=off  T_nominal_unit=K  T_nominal_value=1  Q_specify=off  Q_priority=High  Q=0 J/s  Q_nominal_specify=off  Q_nominal_unit=W  Q_nominal_value=1
  Air-roof convection : fl_lib/Thermal/Thermal Elements/Convective Heat Transfer  thermal_type=foundation.enum.constant_variable.constant  area=area_roof_room3 m^2  heat_tr_coeff=h_air_roof W/(m^2 * K)  min_heat_tr_coeff=1e-3 W/(K*m^2)  T_specify=off  T_priority=None  T=0 K  T_nominal_specify=off  T_nominal_unit=K  T_nominal_value=1  Q_specify=off  Q_priority=None  Q=0 J/s  Q_nominal_specify=off  Q_nominal_unit=W  Q_nominal_value=1
  Air-wall convection : fl_lib/Thermal/Thermal Elements/Convective Heat Transfer  thermal_type=foundation.enum.constant_variable.constant  area=area_wall_room3 m^2  heat_tr_coeff=h_air_wall W/(m^2 * K)  min_heat_tr_coeff=1e-3 W/(K*m^2)  T_specify=off  T_priority=None  T=0 K  T_nominal_specify=off  T_nominal_unit=K  T_nominal_value=1  Q_specify=off  Q_priority=None  Q=0 J/s  Q_nominal_specify=off  Q_nominal_unit=W  Q_nominal_value=1
  Air-window convection : fl_lib/Thermal/Thermal Elements/Convective Heat Transfer  thermal_type=foundation.enum.constant_variable.constant  area=area_window_room3 m^2  heat_tr_coeff=h_air_window W/(m^2 * K)  min_heat_tr_coeff=1e-3 W/(K*m^2)  T_specify=off  T_priority=None  T=0 K  T_nominal_specify=off  T_nominal_unit=K  T_nominal_value=1  Q_specify=off  Q_priority=None  Q=0 J/s  Q_nominal_specify=off  Q_nominal_unit=W  Q_nominal_value=1
  Half roof-air conduction : fl_lib/Thermal/Thermal Elements/Conductive Heat Transfer  thermal_type=foundation.enum.ConstantVariableTabulated.Constant  wall_geometry=foundation.enum.ConductionWallGeometry.Planar  area=area_roof_room3 m^2  thickness=LRoof/2 m  d_in=0.05 m  d_out=0.1 m  L=1 m  th_cond_min=10 W/(K*m)  th_cond=kRoof W/(m*K)  th_cond_TLU=[413, 401, 392, 383, 371, 357, 342] W/(K*m)  temp_TLU=[200, 273, 400, 600, 800, 1000, 1200] K  T_specify=off  T_priority=None  T=0 K  T_nominal_specify=off  T_nominal_unit=K  T_nominal_value=1  Q_specify=off  Q_priority=None  Q=0 J/s  Q_nominal_specify=off  Q_nominal_unit=W  Q_nominal_value=1
  Half roof-atmosphere conduction : fl_lib/Thermal/Thermal Elements/Conductive Heat Transfer  thermal_type=foundation.enum.ConstantVariableTabulated.Constant  wall_geometry=foundation.enum.ConductionWallGeometry.Planar  area=area_roof_room3 m^2  thickness=LRoof/2 m  d_in=0.05 m  d_out=0.1 m  L=1 m  th_cond_min=10 W/(K*m)  th_cond=kRoof W/(m*K)  th_cond_TLU=[413, 401, 392, 383, 371, 357, 342] W/(K*m)  temp_TLU=[200, 273, 400, 600, 800, 1000, 1200] K  T_specify=off  T_priority=None  T=0 K  T_nominal_specify=off  T_nominal_unit=K  T_nominal_value=1  Q_specify=off  Q_priority=None  Q=0 J/s  Q_nominal_specify=off  Q_nominal_unit=W  Q_nominal_value=1
  Half wall-air conduction : fl_lib/Thermal/Thermal Elements/Conductive Heat Transfer  thermal_type=foundation.enum.ConstantVariableTabulated.Constant  wall_geometry=foundation.enum.ConductionWallGeometry.Planar  area=area_wall_room3 m^2  thickness=LWall/2 m  d_in=0.05 m  d_out=0.1 m  L=1 m  th_cond_min=10 W/(K*m)  th_cond=kWall W/(m*K)  th_cond_TLU=[413, 401, 392, 383, 371, 357, 342] W/(K*m)  temp_TLU=[200, 273, 400, 600, 800, 1000, 1200] K  T_specify=off  T_priority=None  T=0 K  T_nominal_specify=off  T_nominal_unit=K  T_nominal_value=1  Q_specify=off  Q_priority=None  Q=0 J/s  Q_nominal_specify=off  Q_nominal_unit=W  Q_nominal_value=1
  Half wall-atmosphere conduction : fl_lib/Thermal/Thermal Elements/Conductive Heat Transfer  thermal_type=foundation.enum.ConstantVariableTabulated.Constant  wall_geometry=foundation.enum.ConductionWallGeometry.Planar  area=area_wall_room3 m^2  thickness=LWall/2 m  d_in=0.05 m  d_out=0.1 m  L=1 m  th_cond_min=10 W/(K*m)  th_cond=kWall W/(m*K)  th_cond_TLU=[413, 401, 392, 383, 371, 357, 342] W/(K*m)  temp_TLU=[200, 273, 400, 600, 800, 1000, 1200] K  T_specify=off  T_priority=None  T=0 K  T_nominal_specify=off  T_nominal_unit=K  T_nominal_value=1  Q_specify=off  Q_priority=None  Q=0 J/s  Q_nominal_specify=off  Q_nominal_unit=W  Q_nominal_value=1
  Half window-air conduction : fl_lib/Thermal/Thermal Elements/Conductive Heat Transfer  thermal_type=foundation.enum.ConstantVariableTabulated.Constant  wall_geometry=foundation.enum.ConductionWallGeometry.Planar  area=area_window_room3 m^2  thickness=LWindow/2 m  d_in=0.05 m  d_out=0.1 m  L=1 m  th_cond_min=10 W/(K*m)  th_cond=kWindow W/(m*K)  th_cond_TLU=[413, 401, 392, 383, 371, 357, 342] W/(K*m)  temp_TLU=[200, 273, 400, 600, 800, 1000, 1200] K  T_specify=off  T_priority=None  T=0 K  T_nominal_specify=off  T_nominal_unit=K  T_nominal_value=1  Q_specify=off  Q_priority=None  Q=0 J/s  Q_nominal_specify=off  Q_nominal_unit=W  Q_nominal_value=1
  Half window-atmosphere conduction : fl_lib/Thermal/Thermal Elements/Conductive Heat Transfer  thermal_type=foundation.enum.ConstantVariableTabulated.Constant  wall_geometry=foundation.enum.ConductionWallGeometry.Planar  area=area_window_room3 m^2  thickness=LWindow/2 m  d_in=0.05 m  d_out=0.1 m  L=1 m  th_cond_min=10 W/(K*m)  th_cond=kWindow W/(m*K)  th_cond_TLU=[413, 401, 392, 383, 371, 357, 342] W/(K*m)  temp_TLU=[200, 273, 400, 600, 800, 1000, 1200] K  T_specify=off  T_priority=None  T=0 K  T_nominal_specify=off  T_nominal_unit=K  T_nominal_value=1  Q_specify=off  Q_priority=None  Q=0 J/s  Q_nominal_specify=off  Q_nominal_unit=W  Q_nominal_value=1
  Roof thermal mass : fl_lib/Thermal/Thermal Elements/Thermal Mass  mass_type=foundation.enum.constant_variable.constant  mass=area_roof_room3*LRoof*roofDensity kg  sp_heat=c_roof J/kg/K  mass_min=1e-6 kg  num_ports=foundation.enum.numPorts2.one  m_specify=off  m_priority=High  m=1 kg  m_nominal_specify=off  m_nominal_unit=kg  m_nominal_value=1  T_specify=on  T_priority=High  T=20 degC  T_nominal_specify=off  T_nominal_unit=K  T_nominal_value=1  Q_specify=off  Q_priority=None  Q=0 J/s  Q_nominal_specify=off  Q_nominal_unit=W  Q_nominal_value=1
  Roof-atmosphere convection : fl_lib/Thermal/Thermal Elements/Convective Heat Transfer  thermal_type=foundation.enum.constant_variable.constant  area=area_roof_room3 m^2  heat_tr_coeff=h_roof_atm W/(m^2 * K)  min_heat_tr_coeff=1e-3 W/(K*m^2)  T_specify=off  T_priority=None  T=0 K  T_nominal_specify=off  T_nominal_unit=K  T_nominal_value=1  Q_specify=off  Q_priority=None  Q=0 J/s  Q_nominal_specify=off  Q_nominal_unit=W  Q_nominal_value=1
  Roof-atmosphere leakage : fl_lib/Thermal/Thermal Elements/Convective Heat Transfer  thermal_type=foundation.enum.constant_variable.constant  area=area_roof_room3*leak_roof_percent m^2  heat_tr_coeff=h_roof_atm W/(m^2 * K)  min_heat_tr_coeff=1e-3 W/(K*m^2)  T_specify=off  T_priority=None  T=0 K  T_nominal_specify=off  T_nominal_unit=K  T_nominal_value=1  Q_specify=off  Q_priority=None  Q=0 J/s  Q_nominal_specify=off  Q_nominal_unit=W  Q_nominal_value=1
  Simulink-PS Converter : nesl_utility/Simulink-PS Converter  PhysicalDomain=network_engine_domain  SubClassName=ps_input  LeftPortType=input  RightPortType=output  PseudoPeriodic=off  Frequencies=[]  NoiseDistribution=none  NoiseParameters=[]  Unit=degC  AffineConversion=on  FilteringAndDerivatives=zero  SimscapeFilterOrder=1  InputFilterTimeConstant=.001  UdotUserProvided=1
  TRef : fl_lib/Thermal/Thermal Elements/Thermal Reference
  Temperature source atmosphere : fl_lib/Thermal/Thermal Sources/Controlled Temperature Source
  Temperature sensor : Subsystem
  Wall thermal mass : fl_lib/Thermal/Thermal Elements/Thermal Mass  mass_type=foundation.enum.constant_variable.constant  mass=area_wall_room3 * LWall * wallDensity kg  sp_heat=c_wall J/kg/K  mass_min=1e-6 kg  num_ports=foundation.enum.numPorts2.one  m_specify=off  m_priority=High  m=1 kg  m_nominal_specify=off  m_nominal_unit=kg  m_nominal_value=1  T_specify=on  T_priority=High  T=20 degC  T_nominal_specify=off  T_nominal_unit=K  T_nominal_value=1  Q_specify=off  Q_priority=None  Q=0 J/s  Q_nominal_specify=off  Q_nominal_unit=W  Q_nominal_value=1
  Wall-atmosphere convection : fl_lib/Thermal/Thermal Elements/Convective Heat Transfer  thermal_type=foundation.enum.constant_variable.constant  area=area_wall_room3 m^2  heat_tr_coeff=h_wall_atm W/(m^2 * K)  min_heat_tr_coeff=1e-3 W/(K*m^2)  T_specify=off  T_priority=None  T=0 K  T_nominal_specify=off  T_nominal_unit=K  T_nominal_value=1  Q_specify=off  Q_priority=None  Q=0 J/s  Q_nominal_specify=off  Q_nominal_unit=W  Q_nominal_value=1
  Wall_atmosphere leakage : fl_lib/Thermal/Thermal Elements/Convective Heat Transfer  thermal_type=foundation.enum.constant_variable.constant  area=area_wall_room3*leak_wall_percent m^2  heat_tr_coeff=h_wall_atm W/(m^2 * K)  min_heat_tr_coeff=1e-3 W/(K*m^2)  T_specify=off  T_priority=None  T=0 K  T_nominal_specify=off  T_nominal_unit=K  T_nominal_value=1  Q_specify=off  Q_priority=None  Q=0 J/s  Q_nominal_specify=off  Q_nominal_unit=W  Q_nominal_value=1
  Window thermal mass : fl_lib/Thermal/Thermal Elements/Thermal Mass  mass_type=foundation.enum.constant_variable.constant  mass=area_window_room3 * LWindow * windowDensity kg  sp_heat=c_window J/kg/K  mass_min=1e-6 kg  num_ports=foundation.enum.numPorts2.one  m_specify=off  m_priority=High  m=1 kg  m_nominal_specify=off  m_nominal_unit=kg  m_nominal_value=1  T_specify=on  T_priority=High  T=20 degC  T_nominal_specify=off  T_nominal_unit=K  T_nominal_value=1  Q_specify=off  Q_priority=None  Q=0 J/s  Q_nominal_specify=off  Q_nominal_unit=W  Q_nominal_value=1
  Window-atmosphere convection : fl_lib/Thermal/Thermal Elements/Convective Heat Transfer  thermal_type=foundation.enum.constant_variable.constant  area=area_window_room3 m^2  heat_tr_coeff=h_window_atm W/(m^2 * K)  min_heat_tr_coeff=1e-3 W/(K*m^2)  T_specify=off  T_priority=None  T=0 K  T_nominal_specify=off  T_nominal_unit=K  T_nominal_value=1  Q_specify=off  Q_priority=None  Q=0 J/s  Q_nominal_specify=off  Q_nominal_unit=W  Q_nominal_value=1
  Window-atmosphere leakage : fl_lib/Thermal/Thermal Elements/Convective Heat Transfer  thermal_type=foundation.enum.constant_variable.constant  area=area_window_room3*leak_win_percent m^2  heat_tr_coeff=h_window_atm W/(m^2 * K)  min_heat_tr_coeff=1e-3 W/(K*m^2)  T_specify=off  T_priority=None  T=0 K  T_nominal_specify=off  T_nominal_unit=K  T_nominal_value=1  Q_specify=off  Q_priority=None  Q=0 J/s  Q_nominal_specify=off  Q_nominal_unit=W  Q_nominal_value=1
  Heater : PMIOPort  Tag=PMCPort  Side=Left
  Troom3 : Outport  VectorParamsAs1DForOutWhenUnconnected=off
  wires:
  Temperature sensor/1(T) -> Troom3/1  "Room3"
  Tatm/1 -> Simulink-PS Converter/1
  connections:
  Air-roof convection/LConn1 -- Air thermal mass/LConn1 -- Air-wall convection/LConn1 -- Air-window convection/LConn1 -- Heater/RConn1 -- Temperature sensor/LConn1
  Wall thermal mass/LConn1 -- Half wall-atmosphere conduction/LConn1 -- Half wall-air conduction/RConn1
  Window thermal mass/LConn1 -- Half window-atmosphere conduction/LConn1 -- Half window-air conduction/RConn1
  Half roof-air conduction/RConn1 -- Half roof-atmosphere conduction/LConn1 -- Roof thermal mass/LConn1
  Half wall-air conduction/LConn1 -- Air-wall convection/RConn1 -- Wall_atmosphere leakage/LConn1
  Air-window convection/RConn1 -- Window-atmosphere leakage/LConn1 -- Half window-air conduction/LConn1
  Half roof-air conduction/LConn1 -- Air-roof convection/RConn1 -- Roof-atmosphere leakage/LConn1
  TRef/LConn1 -- Temperature source atmosphere/RConn2
  Wall-atmosphere convection/LConn1 -- Half wall-atmosphere conduction/RConn1
  Half roof-atmosphere conduction/RConn1 -- Roof-atmosphere convection/LConn1
  Window-atmosphere convection/LConn1 -- Half window-atmosphere conduction/RConn1
  Temperature source atmosphere/RConn1 -- Simulink-PS Converter/RConn1
  Wall-atmosphere convection/RConn1 -- Window-atmosphere leakage/RConn1 -- Window-atmosphere convection/RConn1 -- Roof-atmosphere convection/RConn1 -- Roof-atmosphere leakage/RConn1 -- Wall_atmosphere leakage/RConn1 -- Temperature source atmosphere/LConn1
